simulink subsystem "driveControl_Component"  (R2023a)
settings: Solver=VariableStepAuto  StartTime=0.0  StopTime=10.0  RelTol=1e-3
settings Model: Creator=Franz  LastModifiedBy=Franz

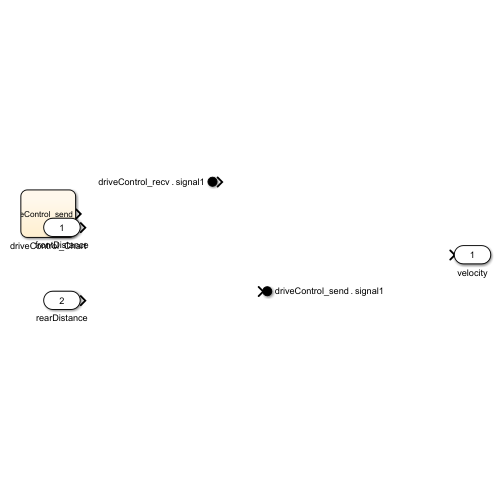
[thumbnail: Simulink's stored preview of the top-level diagram]
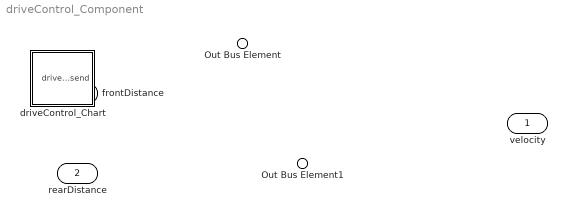
== system driveControl_Component ==
  frontDistance : Inport
  rearDistance : Inport  Port=2
  Out Bus Element : Inport  Port=3  PortName=driveControl_recv  Element=signal1
  driveControl_Chart : Stateflow chart  TreatAsAtomicUnit=on
  velocity : Outport
  Out Bus Element1 : Outport  Port=2  PortName=driveControl_send  Element=signal1

== stateflow chart driveControl_Component/driveControl_Chart ==
  state chart
    state chartRegion [parallel]
      settings: executionOrder=1
      state DriveControlComponent
        state driveControlPort [parallel]
          settings: executionOrder=1
          state Idle
          state WaitforCoordinator
          state WaitForOvertaking
          (default) -> Idle
          WaitForOvertaking -> Idle : [communicator_recv == 2]{send(executedOvertaking.overtakingInitPort);}
          WaitforCoordinator -> WaitForOvertaking [order 2] : grantPermission{communicator_send = 1;}
          WaitforCoordinator -> Idle [order 1] : denyPermission{communicator_send = 4;}
          Idle -> WaitforCoordinator : [communicator_recv==1]{send(OvertakingRequested,overtkingIniPort), coordination_Successfull = true;}
        state driving [parallel]
          settings: executionOrder=2
      (default) -> DriveControlComponent
  (default) -> chart
  data: driveControl_send output; frontDistance local Int32; communicator_send local; grantPermission local; coordination_Successfull local
  events: denyPermission local FUNCTION_CALL_EVENT; OvertakingRequested local FUNCTION_CALL_EVENT; communicator_recv local FUNCTION_CALL_EVENT
